simulink model "Template_Matching_Continuous"  (R2020a)
settings: Solver=VariableStepAuto  StartTime=0.0  StopTime=40  RelTol=1e-3
libraries: simulink x1, dspfdesign x1
settings Model: Creator=sbuccelli  LastModifiedBy=diflo

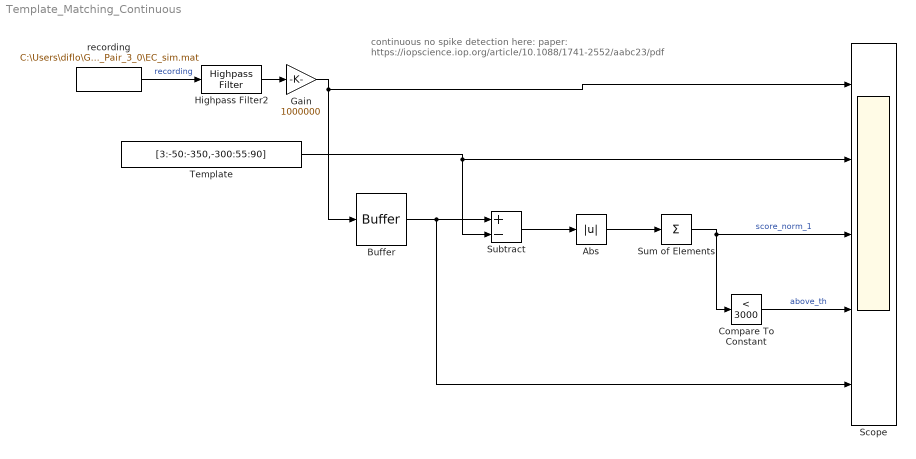
== system Template_Matching_Continuous ==
  note: continuous no spike detection here:
      | paper: https://iopscience.iop.org/article/10.1088/1741-2552/aabc23/pdf
  Abs : Abs
  Buffer : Buffer  N=16  V=15  OutputFrames=off
  Compare To Constant : simulink/Logic and Bit Operations/Compare To Constant  relop=<  const=3000  OutDataTypeStr=boolean
  Gain : Gain  Gain=1000000
  Highpass Filter2 : dspfdesign/Highpass Filter  FilterType=IIR  DesignForMinimumOrder=off  FilterOrder=3  StopbandFrequency=1  PassbandFrequency=300  StopbandAttenuation=80  PassbandRipple=0.1  InheritSampleRate=off  SampleRate=30000  SimulateUsing=Interpreted execution  roundingMode=Floor  coeffsDataTypeStr=fixdt(1,16)
  Scope : Scope  NumInputPorts=5
  Subtract : Sum  Inputs=+-
  Sum of Elements : Sum  Inputs=+
  Template : Constant  Value=[3:-50:-350,-300:55:90]  SampleTime=1/30000
  recording : FromFile  FileName=C:\Users\diflo\Google Drive\IIT - Neuroengineering\MathWorks Project\Data\KampffLab\2014_11_25_Pair_3_0\EC_sim.mat  SampleTime=1/30000
  wires:
  recording/1 -> Highpass Filter2/1  "recording"
  Buffer/1 -> Scope/5, Subtract/1
  Subtract/1 -> Abs/1
  Abs/1 -> Sum of Elements/1
  Sum of Elements/1 -> Compare To Constant/1, Scope/3  "score_norm_1"
  Template/1 -> Subtract/2, Scope/2
  Compare To Constant/1 -> Scope/4  "above_th"
  Gain/1 -> Buffer/1, Scope/1
  Highpass Filter2/1 -> Gain/1
